simulink model "banlance_Car"  (R2023b)
settings: Solver=VariableStepAuto  StartTime=0.0  StopTime=10.0  RelTol=1e-3
settings Model: Creator=xjtu  LastModifiedBy=xjtu

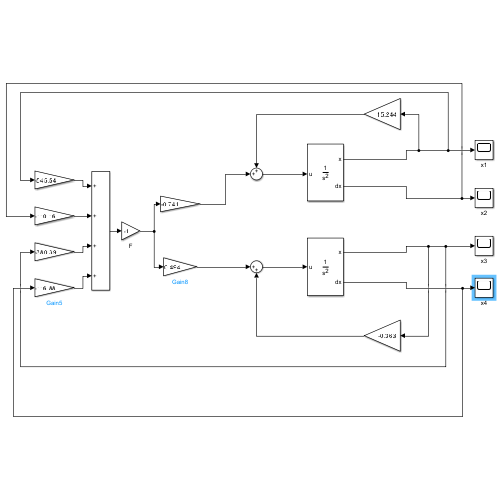
[thumbnail: Simulink's stored preview of the top-level diagram]
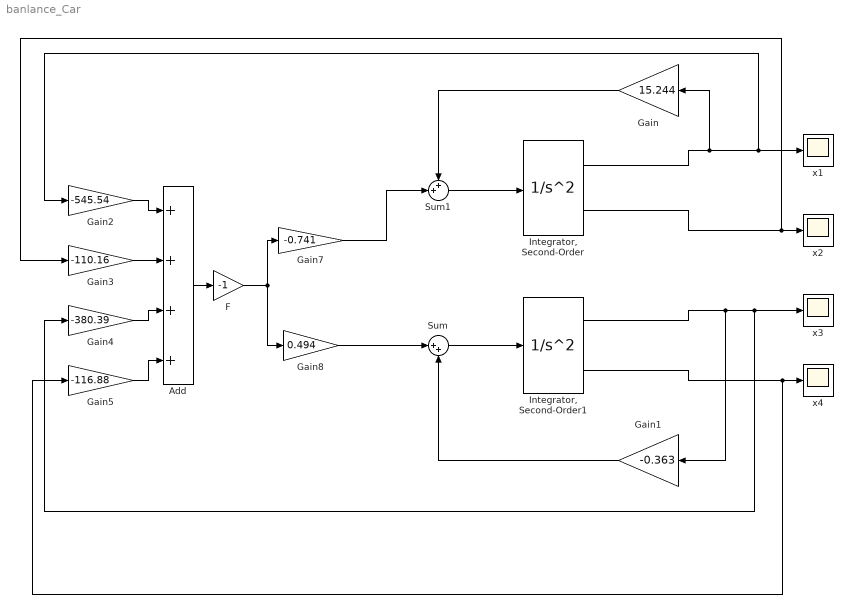
== system banlance_Car ==
  Add : Sum  Inputs=++++
  F : Gain  Gain=-1
  Gain : Gain  Gain=15.244
  Gain1 : Gain  Gain=-0.363
  Gain2 : Gain  Gain=-545.54
  Gain3 : Gain  Gain=-110.16
  Gain4 : Gain  Gain=-380.39
  Gain5 : Gain  Gain=-116.88
  Gain7 : Gain  Gain=-0.741
  Gain8 : Gain  Gain=0.494
  "Integrator, Second-Order" : SecondOrderIntegrator  ICX=1
  "Integrator, Second-Order1" : SecondOrderIntegrator
  Sum : Sum  Inputs=|++
  Sum1 : Sum  Inputs=++|
  x{1..4} (4 alike) : Scope
  wires:
  "Integrator, Second-Order1"/1 -> Gain1/1, Gain4/1, x3/1
  "Integrator, Second-Order1"/2 -> Gain5/1, x4/1
  "Integrator, Second-Order"/2 -> Gain3/1, x2/1
  Sum/1 -> "Integrator, Second-Order1"/1
  Sum1/1 -> "Integrator, Second-Order"/1
  Gain1/1 -> Sum/2
  Gain/1 -> Sum1/1
  Gain2/1 -> Add/1
  Gain3/1 -> Add/2
  Gain4/1 -> Add/3
  Gain5/1 -> Add/4
  Add/1 -> F/1
  F/1 -> Gain8/1, Gain7/1
  Gain7/1 -> Sum1/2
  Gain8/1 -> Sum/1
  "Integrator, Second-Order"/1 -> Gain/1, Gain2/1, x1/1
